simulink model "simple"  (R2021b)
settings: Solver=VariableStepAuto  StartTime=0.0  StopTime=10.0  RelTol=1e-3
settings Model: Creator=anton  LastModifiedBy=anton

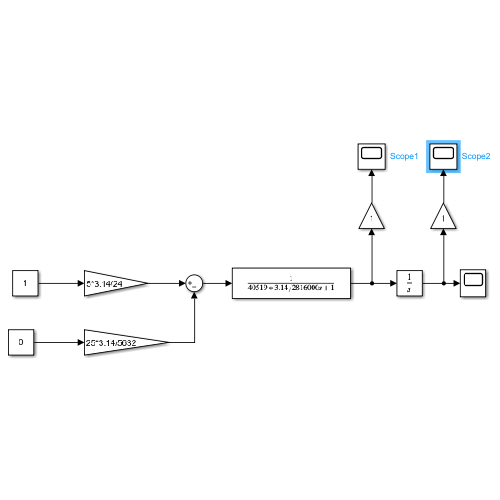
[thumbnail: Simulink's stored preview of the top-level diagram]
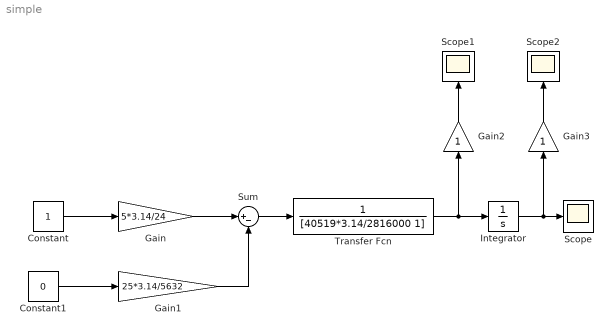
== system simple ==
  Constant : Constant
  Constant1 : Constant  Value=0
  Gain : Gain  Gain=5*3.14/24
  Gain1 : Gain  Gain=25*3.14/5632
  Gain2 : Gain
  Gain3 : Gain
  Integrator : Integrator
  Scope : Scope
  Scope1 : Scope
  Scope2 : Scope
  Sum : Sum  Inputs=|+-
  Transfer Fcn : TransferFcn  Denominator=[40519*3.14/2816000 1]
  wires:
  Constant/1 -> Gain/1
  Gain/1 -> Sum/1
  Constant1/1 -> Gain1/1
  Gain1/1 -> Sum/2
  Sum/1 -> Transfer Fcn/1
  Transfer Fcn/1 -> Gain2/1, Integrator/1
  Integrator/1 -> Gain3/1, Scope/1
  Gain2/1 -> Scope1/1
  Gain3/1 -> Scope2/1
